simulink model "DSB_SC"  (R2020b)
settings: Solver=VariableStepAuto  StartTime=0.0  StopTime=10.0  RelTol=1e-3
libraries: dsparch4 x1
settings Model: Creator=taone  LastModifiedBy=htn
settings SFSimCC: CustomCodeUndefinedFunction=UseInterfaceOnly

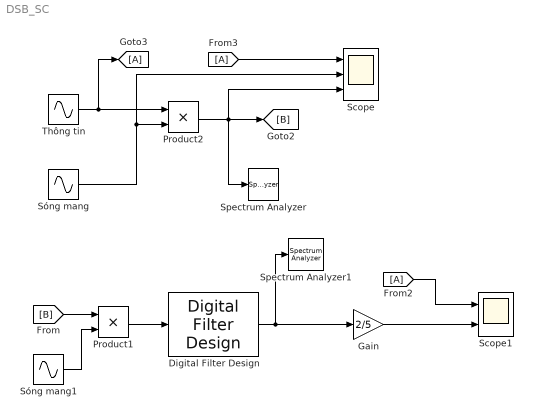
== system DSB_SC ==
  Digital Filter Design : dsparch4/Digital Filter Design  mwdsp_browser_bugfix_var=off
  Gain : Gain  Gain=2/5
  Product1 : Product
  Product2 : Product
  Scope : Scope  NumInputPorts=3
  Scope1 : Scope  NumInputPorts=2
  Spectrum Analyzer : SpectrumAnalyzer
  Spectrum Analyzer1 : SpectrumAnalyzer
  Sóng mang : Sin  Amplitude=5  Frequency=2*pi*5000  SampleTime=1/80000
  Sóng mang1 : Sin  Frequency=2*pi*5000  SampleTime=1/80000
  Thông tin : Sin  Frequency=2*pi*200  SampleTime=1/80000
  wires:
  [A] -> Scope/1
  Product1/1 -> Digital Filter Design/1
  Sóng mang1/1 -> Product1/2
  [B] -> Product1/1
  Digital Filter Design/1 -> Gain/1, Spectrum Analyzer1/1
  Product2/1 -> Spectrum Analyzer/1, Scope/3, [B]
  Thông tin/1 -> Product2/1, [A]
  Sóng mang/1 -> Scope/2, Product2/2
  Gain/1 -> Scope1/2
  [A] -> Scope1/1
